simulink model "motor_speed_control"  (R2017a)
settings: Solver=ode45  StartTime=0.0  StopTime=40  RelTol=1e-3  EnableMultiTasking=on
values from neighbouring files (symbols this model uses):
  B = 2.8645e-05    [parameters.m]
  I = Irt+Iw    (= 0.000113883308987)    [parameters.m]
  Ki_current = 10    [currentController.m]
  Ki_speed = 40    [speedController.m]
  KM = 0.09    [parameters.m]
  Kp_current = 13.961    [currentController.m]
  Kp_speed = 5    [speedController.m]
  Kv = 0.012    [parameters.m]
  L = (5e-4)*2    (= 0.001)    [parameters.m]
  R = 2*Rfn    (= 3.8)    [parameters.m]
  rad2rpm = 60/(2*pi)    (= 9.54929658551)    [parameters.m]
settings Model: Creator=root  LastModifiedBy=gdiazh
settings DataIOCC: LimitDataPoints=on  SaveFormat=Array  SignalLoggingSaveFormat=ModelDataLogs
settings OptimizationCC: ExpressionDepthLimit=2147483647  LifeSpan=inf
settings DebuggingCC: UnderspecifiedInitializationDetection=Classic  MergeDetectMultiDrivingBlocksExec=none  SolverPrmCheckMsg=warning  FcnCallInpInsideContextMsg=warning  StateNameClashWarn=warning  SFUnexpectedBacktrackingDiag=warning  SFNoUnconditionalDefaultTransitionDiag=warning  SFExecutionAtInitializationDiag=none
settings HardwareCC: ProdBitPerPointer=32  ProdBitPerSizeT=32  ProdBitPerPtrDiffT=32  ProdLargestAtomicFloat=None  ProdIntDivRoundTo=Undefined  ProdEndianess=Unspecified  ProdWordSize=32  ProdHWDeviceType=32-bit Generic
settings ModelReferenceCC: PropagateSignalLabelsOutOfModel=off
settings GRTTargetCC: TargetLangStandard=C89/C90 (ANSI)  GeneratePreprocessorConditionals=Disable all
settings ConfigComp: CovMetricSettings=dw  CovHtmlReporting=on  CovSaveCumulativeToWorkspaceVar=on  CovSaveSingleToWorkspaceVar=on  CovExternalEMLEnable=off

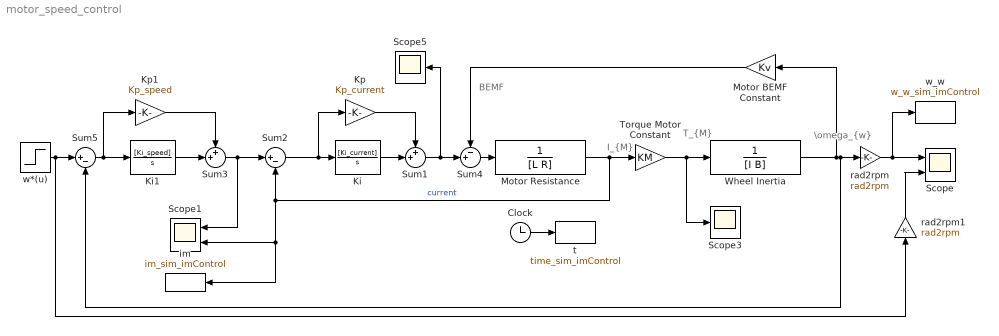
== system motor_speed_control ==
  note: T_{M}
  note: I_{M}
  note: BEMF
  note: \omega_{w}
  Clock : Clock
  Ki : TransferFcn  Numerator=[Ki_current]  Denominator=[1 0]
  Ki1 : TransferFcn  Numerator=[Ki_speed]  Denominator=[1 0]
  Kp : Gain  Gain=Kp_current
  Kp1 : Gain  Gain=Kp_speed
  Motor BEMF Constant : Gain  Gain=Kv
  Motor Resistance : TransferFcn  Denominator=[L R]
  Scope : Scope  NumInputPorts=2
  Scope1 : Scope  NumInputPorts=2
  Scope3 : Scope
  Scope5 : Scope
  Sum1 : Sum  Inputs=++|
  Sum2 : Sum  Inputs=|+-
  Sum3 : Sum  Inputs=++|
  Sum4 : Sum  Inputs=-+|
  Sum5 : Sum  Inputs=|+-
  Torque Motor Constant : Gain  Gain=KM
  Wheel Inertia : TransferFcn  Denominator=[I B]
  im : ToWorkspace  VariableName=im_sim_imControl  SampleTime=-1
      settings: Save2DSignal=2-D array (concatenate along first dimension)
  rad2rpm : Gain  Gain=rad2rpm
  rad2rpm1 : Gain  Gain=rad2rpm
  t : ToWorkspace  VariableName=time_sim_imControl  SampleTime=-1
      settings: Save2DSignal=2-D array (concatenate along first dimension)
  w*(u) : Step  Time=2  After=100  SampleTime=0
  w_w : ToWorkspace  VariableName=w_w_sim_imControl  SampleTime=-1
      settings: Save2DSignal=2-D array (concatenate along first dimension)
  wires:
  Sum4/1 -> Motor Resistance/1
  Motor Resistance/1 -> Torque Motor Constant/1, im/1, Scope1/2, Sum2/2  "current"
  Torque Motor Constant/1 -> Wheel Inertia/1, Scope3/1
  Motor BEMF Constant/1 -> Sum4/1
  rad2rpm/1 -> w_w/1, Scope/1
  Clock/1 -> t/1
  Ki/1 -> Sum1/2
  Kp/1 -> Sum1/1
  Sum1/1 -> Scope5/1, Sum4/2
  Sum2/1 -> Kp/1, Ki/1
  Sum3/1 -> Scope1/1, Sum2/1
  Ki1/1 -> Sum3/2
  Kp1/1 -> Sum3/1
  Sum5/1 -> Kp1/1, Ki1/1
  w*(u)/1 -> rad2rpm1/1, Sum5/1
  Wheel Inertia/1 -> Sum5/2, rad2rpm/1, Motor BEMF Constant/1
  rad2rpm1/1 -> Scope/2
